simulink model "TST_ActMod_Q2Trq"  (R2016b)
settings: Solver=FixedStepDiscrete  StartTime=0.0  StopTime=simTime  FixedStep=sampleTime  RelTol=1e-3
values from neighbouring files (symbols this model uses):
  testCase = 1    [initTST_ActMod_Q2Trq_001.m]    (also in initTST_ActMod_Q2Trq_002.m = 2)
libraries: simulink x5, UnitTest_Lib x2
settings Model: Creator=zhengjinyan  LastModifiedBy=zhengjinyan
settings DebuggingCC: SignalRangeChecking=error

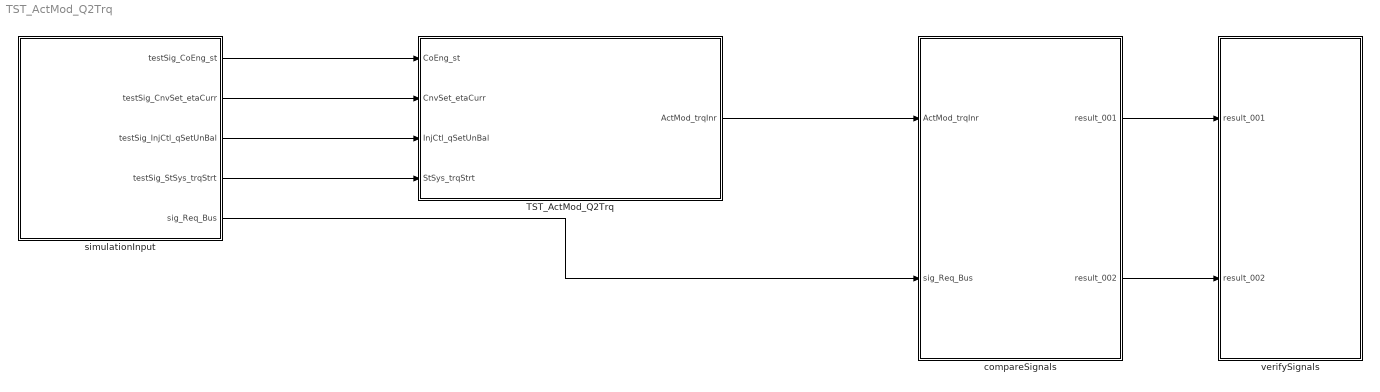
== system TST_ActMod_Q2Trq ==
  TST_ActMod_Q2Trq : Subsystem
  compareSignals : Subsystem
  simulationInput : Subsystem
  verifySignals : Subsystem
  wires:
  simulationInput/1(testSig_CoEng_st) -> TST_ActMod_Q2Trq/1(CoEng_st)
  simulationInput/2(testSig_CnvSet_etaCurr) -> TST_ActMod_Q2Trq/2(CnvSet_etaCurr)
  simulationInput/3(testSig_InjCtl_qSetUnBal) -> TST_ActMod_Q2Trq/3(InjCtl_qSetUnBal)
  simulationInput/4(testSig_StSys_trqStrt) -> TST_ActMod_Q2Trq/4(StSys_trqStrt)
  TST_ActMod_Q2Trq/1(ActMod_trqInr) -> compareSignals/1(ActMod_trqInr)
  simulationInput/5(sig_Req_Bus) -> compareSignals/2(sig_Req_Bus)
  compareSignals/1(result_001) -> verifySignals/1(result_001)
  compareSignals/2(result_002) -> verifySignals/2(result_002)

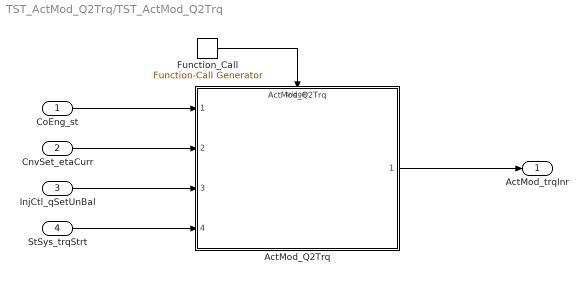
== system TST_ActMod_Q2Trq/TST_ActMod_Q2Trq ==
  CoEng_st : Inport
  CnvSet_etaCurr : Inport  Port=2
  InjCtl_qSetUnBal : Inport  Port=3
  StSys_trqStrt : Inport  Port=4
  ActMod_Q2Trq : ModelReference  ModelNameDialog=ActMod_Q2Trq  SimulationMode=Normal  ModelReferenceVersion=1.2  TriggerPortName=function  TriggerPortTriggerType=function-call  TriggerPortStatesWhenEnabling=held
  Function_Call : simulink/Ports & Subsystems/Function-Call Generator  sample_time=sampleTime  numberOfIterations=1
  ActMod_trqInr : Outport
  wires:
  Function_Call/1 -> ActMod_Q2Trq/Trigger
  CoEng_st/1 -> ActMod_Q2Trq/1
  CnvSet_etaCurr/1 -> ActMod_Q2Trq/2
  InjCtl_qSetUnBal/1 -> ActMod_Q2Trq/3
  StSys_trqStrt/1 -> ActMod_Q2Trq/4
  ActMod_Q2Trq/1 -> ActMod_trqInr/1

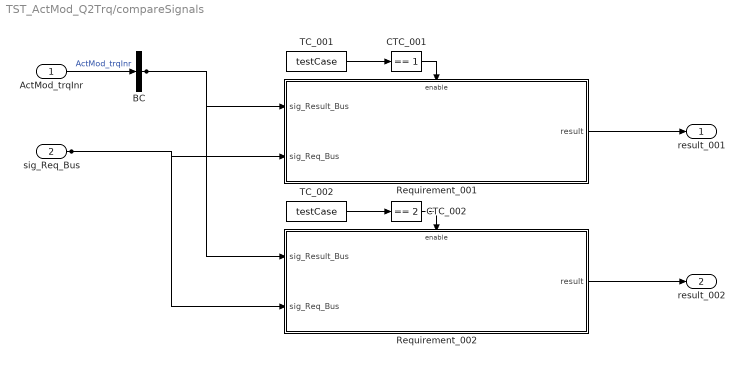
== system TST_ActMod_Q2Trq/compareSignals ==
  ActMod_trqInr : Inport
  sig_Req_Bus : Inport  Port=2
  BC : BusCreator  Inputs=1
  CTC_001 : simulink/Logic and Bit Operations/Compare To Constant  relop===  const=1  OutDataTypeStr=boolean
  CTC_002 : simulink/Logic and Bit Operations/Compare To Constant  relop===  const=2  OutDataTypeStr=boolean
  Requirement_001 : Subsystem
  Requirement_002 : Subsystem
  TC_001 : Constant  Value=testCase
  TC_002 : Constant  Value=testCase
  result_001 : Outport
  result_002 : Outport  Port=2
  wires:
  ActMod_trqInr/1 -> BC/1  "ActMod_trqInr"
  TC_001/1 -> CTC_001/1
  CTC_001/1 -> Requirement_001/Enable
  sig_Req_Bus/1 -> Requirement_001/2(sig_Req_Bus), Requirement_002/2(sig_Req_Bus)
  BC/1 -> Requirement_001/1(sig_Result_Bus), Requirement_002/1(sig_Result_Bus)
  Requirement_001/1(result) -> result_001/1
  TC_002/1 -> CTC_002/1
  CTC_002/1 -> Requirement_002/Enable
  Requirement_002/1(result) -> result_002/1

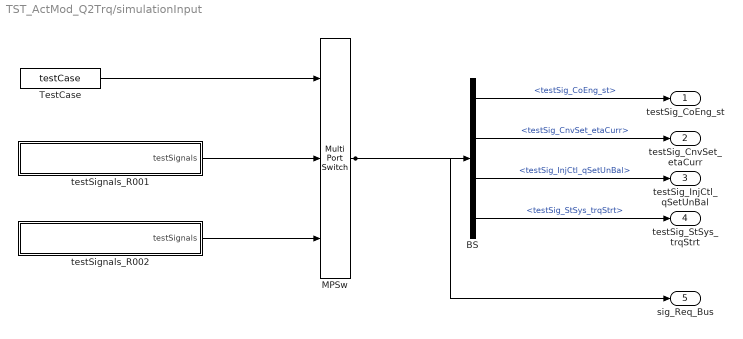
== system TST_ActMod_Q2Trq/simulationInput ==
  BS : BusSelector  OutputSignals=testSig_CoEng_st,testSig_CnvSet_etaCurr,testSig_InjCtl_qSetUnBal,testSig_StSys_trqStrt
  MPSw : MultiPortSwitch  Inputs=2  SaturateOnIntegerOverflow=on  InputSameDT=on
  TestCase : Constant  Value=testCase
  testSignals_R001 : Subsystem
  testSignals_R002 : Subsystem
  testSig_CoEng_st : Outport
  testSig_CnvSet_etaCurr : Outport  Port=2
  testSig_InjCtl_qSetUnBal : Outport  Port=3
  testSig_StSys_trqStrt : Outport  Port=4
  sig_Req_Bus : Outport  Port=5
  wires:
  BS/1 -> testSig_CoEng_st/1  "<testSig_CoEng_st>"
  BS/2 -> testSig_CnvSet_etaCurr/1  "<testSig_CnvSet_etaCurr>"
  BS/3 -> testSig_InjCtl_qSetUnBal/1  "<testSig_InjCtl_qSetUnBal>"
  BS/4 -> testSig_StSys_trqStrt/1  "<testSig_StSys_trqStrt>"
  MPSw/1 -> BS/1, sig_Req_Bus/1
  TestCase/1 -> MPSw/1
  testSignals_R001/1(testSignals) -> MPSw/2
  testSignals_R002/1(testSignals) -> MPSw/3

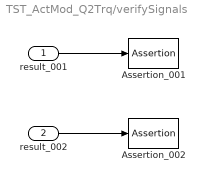
== system TST_ActMod_Q2Trq/verifySignals ==
  result_001 : Inport
  result_002 : Inport  Port=2
  Assertion_001 : Assertion  Enabled=off
  Assertion_002 : Assertion  Enabled=off
  wires:
  result_001/1 -> Assertion_001/1
  result_002/1 -> Assertion_002/1

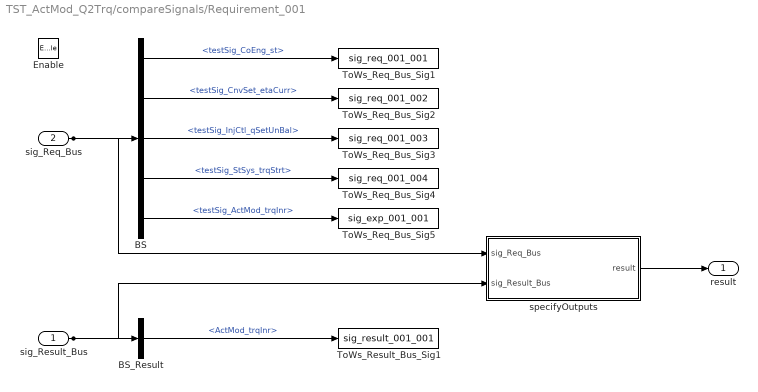
== system TST_ActMod_Q2Trq/compareSignals/Requirement_001 ==
  sig_Result_Bus : Inport
  sig_Req_Bus : Inport  Port=2
  Enable : EnablePort
  BS : BusSelector  OutputSignals=testSig_CoEng_st,testSig_CnvSet_etaCurr,testSig_InjCtl_qSetUnBal,testSig_StSys_trqStrt,testSig_ActMod_trqInr
  BS_Result : BusSelector  OutputSignals=ActMod_trqInr
  ToWs_Req_Bus_Sig1 : ToWorkspace  VariableName=sig_req_001_001  SaveFormat=Structure With Time
  ToWs_Req_Bus_Sig2 : ToWorkspace  VariableName=sig_req_001_002  SaveFormat=Structure With Time
  ToWs_Req_Bus_Sig3 : ToWorkspace  VariableName=sig_req_001_003  SaveFormat=Structure With Time
  ToWs_Req_Bus_Sig4 : ToWorkspace  VariableName=sig_req_001_004  SaveFormat=Structure With Time
  ToWs_Req_Bus_Sig5 : ToWorkspace  VariableName=sig_exp_001_001  SaveFormat=Structure With Time
  ToWs_Result_Bus_Sig1 : ToWorkspace  VariableName=sig_result_001_001  SaveFormat=Structure With Time
  specifyOutputs : Subsystem
  result : Outport
  wires:
  sig_Req_Bus/1 -> BS/1, specifyOutputs/1(sig_Req_Bus)
  BS/1 -> ToWs_Req_Bus_Sig1/1  "<testSig_CoEng_st>"
  BS/2 -> ToWs_Req_Bus_Sig2/1  "<testSig_CnvSet_etaCurr>"
  BS/3 -> ToWs_Req_Bus_Sig3/1  "<testSig_InjCtl_qSetUnBal>"
  BS/4 -> ToWs_Req_Bus_Sig4/1  "<testSig_StSys_trqStrt>"
  BS/5 -> ToWs_Req_Bus_Sig5/1  "<testSig_ActMod_trqInr>"
  sig_Result_Bus/1 -> BS_Result/1, specifyOutputs/2(sig_Result_Bus)
  BS_Result/1 -> ToWs_Result_Bus_Sig1/1  "<ActMod_trqInr>"
  specifyOutputs/1(result) -> result/1

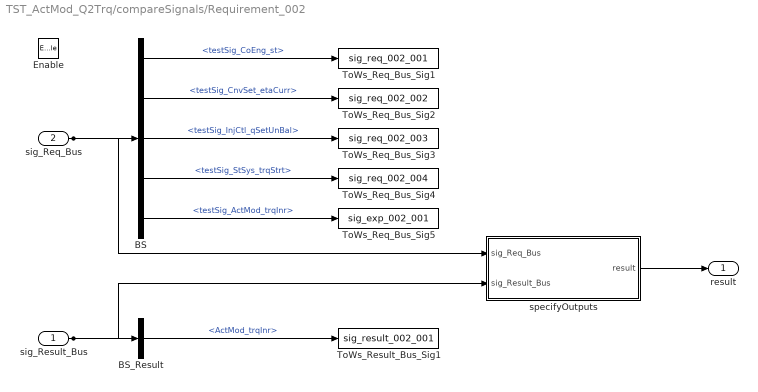
== system TST_ActMod_Q2Trq/compareSignals/Requirement_002 ==
  sig_Result_Bus : Inport
  sig_Req_Bus : Inport  Port=2
  Enable : EnablePort
  BS : BusSelector  OutputSignals=testSig_CoEng_st,testSig_CnvSet_etaCurr,testSig_InjCtl_qSetUnBal,testSig_StSys_trqStrt,testSig_ActMod_trqInr
  BS_Result : BusSelector  OutputSignals=ActMod_trqInr
  ToWs_Req_Bus_Sig1 : ToWorkspace  VariableName=sig_req_002_001  SaveFormat=Structure With Time
  ToWs_Req_Bus_Sig2 : ToWorkspace  VariableName=sig_req_002_002  SaveFormat=Structure With Time
  ToWs_Req_Bus_Sig3 : ToWorkspace  VariableName=sig_req_002_003  SaveFormat=Structure With Time
  ToWs_Req_Bus_Sig4 : ToWorkspace  VariableName=sig_req_002_004  SaveFormat=Structure With Time
  ToWs_Req_Bus_Sig5 : ToWorkspace  VariableName=sig_exp_002_001  SaveFormat=Structure With Time
  ToWs_Result_Bus_Sig1 : ToWorkspace  VariableName=sig_result_002_001  SaveFormat=Structure With Time
  specifyOutputs : Subsystem
  result : Outport
  wires:
  sig_Req_Bus/1 -> BS/1, specifyOutputs/1(sig_Req_Bus)
  BS/1 -> ToWs_Req_Bus_Sig1/1  "<testSig_CoEng_st>"
  BS/2 -> ToWs_Req_Bus_Sig2/1  "<testSig_CnvSet_etaCurr>"
  BS/3 -> ToWs_Req_Bus_Sig3/1  "<testSig_InjCtl_qSetUnBal>"
  BS/4 -> ToWs_Req_Bus_Sig4/1  "<testSig_StSys_trqStrt>"
  BS/5 -> ToWs_Req_Bus_Sig5/1  "<testSig_ActMod_trqInr>"
  sig_Result_Bus/1 -> BS_Result/1, specifyOutputs/2(sig_Result_Bus)
  BS_Result/1 -> ToWs_Result_Bus_Sig1/1  "<ActMod_trqInr>"
  specifyOutputs/1(result) -> result/1

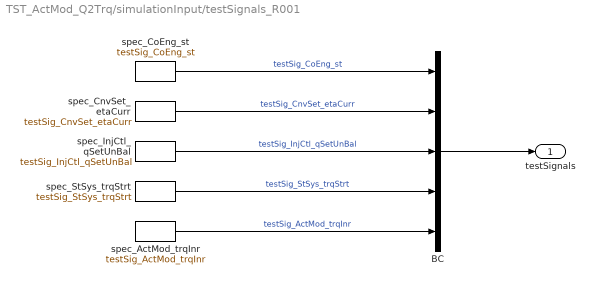
== system TST_ActMod_Q2Trq/simulationInput/testSignals_R001 ==
  BC : BusCreator  Inputs=5
  spec_ActMod_trqInr : FromWorkspace  VariableName=testSig_ActMod_trqInr  Interpolate=off  OutputAfterFinalValue=Holding final value
  spec_CnvSet_etaCurr : FromWorkspace  VariableName=testSig_CnvSet_etaCurr  Interpolate=off  OutputAfterFinalValue=Holding final value
  spec_CoEng_st : FromWorkspace  VariableName=testSig_CoEng_st  Interpolate=off  OutputAfterFinalValue=Holding final value
  spec_InjCtl_qSetUnBal : FromWorkspace  VariableName=testSig_InjCtl_qSetUnBal  Interpolate=off  OutputAfterFinalValue=Holding final value
  spec_StSys_trqStrt : FromWorkspace  VariableName=testSig_StSys_trqStrt  Interpolate=off  OutputAfterFinalValue=Holding final value
  testSignals : Outport
  wires:
  BC/1 -> testSignals/1
  spec_CoEng_st/1 -> BC/1  "testSig_CoEng_st"
  spec_CnvSet_etaCurr/1 -> BC/2  "testSig_CnvSet_etaCurr"
  spec_InjCtl_qSetUnBal/1 -> BC/3  "testSig_InjCtl_qSetUnBal"
  spec_StSys_trqStrt/1 -> BC/4  "testSig_StSys_trqStrt"
  spec_ActMod_trqInr/1 -> BC/5  "testSig_ActMod_trqInr"

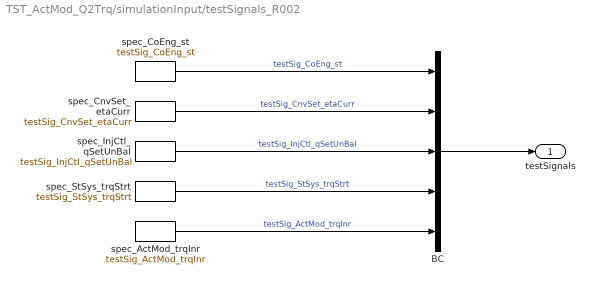
== system TST_ActMod_Q2Trq/simulationInput/testSignals_R002 ==
  BC : BusCreator  Inputs=5
  spec_ActMod_trqInr : FromWorkspace  VariableName=testSig_ActMod_trqInr  Interpolate=off  OutputAfterFinalValue=Holding final value
  spec_CnvSet_etaCurr : FromWorkspace  VariableName=testSig_CnvSet_etaCurr  Interpolate=off  OutputAfterFinalValue=Holding final value
  spec_CoEng_st : FromWorkspace  VariableName=testSig_CoEng_st  Interpolate=off  OutputAfterFinalValue=Holding final value
  spec_InjCtl_qSetUnBal : FromWorkspace  VariableName=testSig_InjCtl_qSetUnBal  Interpolate=off  OutputAfterFinalValue=Holding final value
  spec_StSys_trqStrt : FromWorkspace  VariableName=testSig_StSys_trqStrt  Interpolate=off  OutputAfterFinalValue=Holding final value
  testSignals : Outport
  wires:
  BC/1 -> testSignals/1
  spec_CoEng_st/1 -> BC/1  "testSig_CoEng_st"
  spec_CnvSet_etaCurr/1 -> BC/2  "testSig_CnvSet_etaCurr"
  spec_InjCtl_qSetUnBal/1 -> BC/3  "testSig_InjCtl_qSetUnBal"
  spec_StSys_trqStrt/1 -> BC/4  "testSig_StSys_trqStrt"
  spec_ActMod_trqInr/1 -> BC/5  "testSig_ActMod_trqInr"

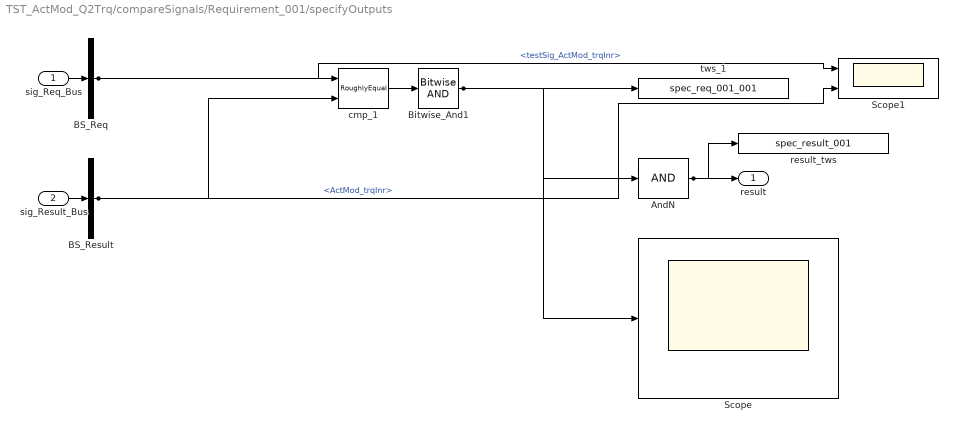
== system TST_ActMod_Q2Trq/compareSignals/Requirement_001/specifyOutputs ==
  sig_Req_Bus : Inport
  sig_Result_Bus : Inport  Port=2
  AndN : Logic  Inputs=1
  BS_Req : BusSelector  OutputSignals=testSig_ActMod_trqInr
  BS_Result : BusSelector  OutputSignals=ActMod_trqInr
  Bitwise_And1 : simulink/Logic and Bit Operations/Bitwise Operator  logicop=AND  UseBitMask=off  BitMask=bin2dec('11011001')  BitMaskRealWorld=Stored Integer
  Scope : Scope
  Scope1 : Scope  NumInputPorts=2
  cmp_1 : UnitTest_Lib/RoughlyEqual  slope=0.1
  result_tws : ToWorkspace  VariableName=spec_result_001
  tws_1 : ToWorkspace  VariableName=spec_req_001_001
  result : Outport
  wires:
  sig_Req_Bus/1 -> BS_Req/1
  sig_Result_Bus/1 -> BS_Result/1
  AndN/1 -> result/1, result_tws/1
  BS_Req/1 -> cmp_1/1, Scope1/1  "<testSig_ActMod_trqInr>"
  BS_Result/1 -> cmp_1/2, Scope1/2  "<ActMod_trqInr>"
  cmp_1/1 -> Bitwise_And1/1
  Bitwise_And1/1 -> tws_1/1, AndN/1, Scope/1

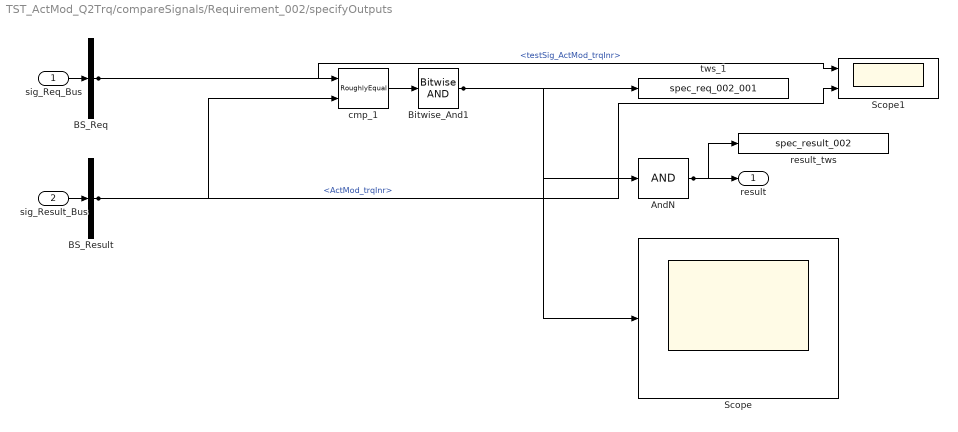
== system TST_ActMod_Q2Trq/compareSignals/Requirement_002/specifyOutputs ==
  sig_Req_Bus : Inport
  sig_Result_Bus : Inport  Port=2
  AndN : Logic  Inputs=1
  BS_Req : BusSelector  OutputSignals=testSig_ActMod_trqInr
  BS_Result : BusSelector  OutputSignals=ActMod_trqInr
  Bitwise_And1 : simulink/Logic and Bit Operations/Bitwise Operator  logicop=AND  UseBitMask=off  BitMask=bin2dec('11011001')  BitMaskRealWorld=Stored Integer
  Scope : Scope
  Scope1 : Scope  NumInputPorts=2
  cmp_1 : UnitTest_Lib/RoughlyEqual  slope=0.1
  result_tws : ToWorkspace  VariableName=spec_result_002
  tws_1 : ToWorkspace  VariableName=spec_req_002_001
  result : Outport
  wires:
  sig_Req_Bus/1 -> BS_Req/1
  sig_Result_Bus/1 -> BS_Result/1
  AndN/1 -> result/1, result_tws/1
  BS_Req/1 -> cmp_1/1, Scope1/1  "<testSig_ActMod_trqInr>"
  BS_Result/1 -> cmp_1/2, Scope1/2  "<ActMod_trqInr>"
  cmp_1/1 -> Bitwise_And1/1
  Bitwise_And1/1 -> tws_1/1, AndN/1, Scope/1
